simulink model "lecture8_mclock"  (Simulink 7.1)
settings: Solver=FixedStepDiscrete  StartTime=0.0  StopTime=Inf  RelTol=1e-3
libraries: simulink x1
settings Model: Creator=pit  LastModifiedBy=pit

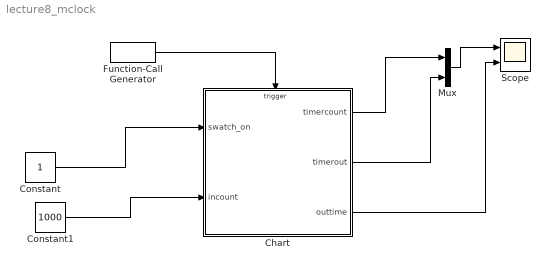
== system lecture8_mclock ==
  Chart : Stateflow chart
  Constant : Constant  OutDataType=sfix(16)  OutScaling=2^0
  Constant1 : Constant  Value=1000  OutDataType=sfix(16)  OutScaling=2^0
  Function-Call Generator : simulink/Ports & Subsystems/Function-Call Generator  sample_time=.05  numberOfIterations=1
  Mux : Mux  Inputs=2
  Scope : Scope  NumInputPorts=2
      settings: YMin=0~84200  YMax=1000~84600
  wires:
  Function-Call Generator/1 -> Chart/Trigger
  Constant/1 -> Chart/1(swatch_on)
  Constant1/1 -> Chart/2(incount)
  Chart/1(timercount) -> Mux/1
  Chart/2(timerout) -> Mux/2
  Mux/1 -> Scope/1
  Chart/3(outtime) -> Scope/2

== stateflow chart Chart ==
  state Off
  state On
    state Timer [parallel]
      settings: executionOrder=1
      state On
        entry:timerout=0
        entry:timercount=incount
        du: timercount=timercount-1
      state Trigger
        entry: timerout=1
      (default) -> On.Timer.On
      On.Timer.On -> Trigger : [timercount<=0]
      Trigger -> On.Timer.On
    state Chrono [parallel]
      entry: outtime=0
      du: outtime=outtime+1
      settings: executionOrder=2
  (default) -> Off
  Off -> On : [swatch_on==1]
  On -> Off : [swatch_on==0]
  data: swatch_on input double; incount input double; timercount output double; timerout output double; outtime output double; count local double
  events: clock input FUNCTION_CALL_EVENT
